simulink model "two_link_inner_loop"  (R2021a)
settings: Solver=VariableStepAuto  StartTime=0.0  StopTime=10.0  RelTol=1e-3
undefined symbols (not defined in the file): a_1, a_2, F, K, K_D, K_F, K_P, M_d, o_r
settings Model: Creator=frida  LastModifiedBy=frida

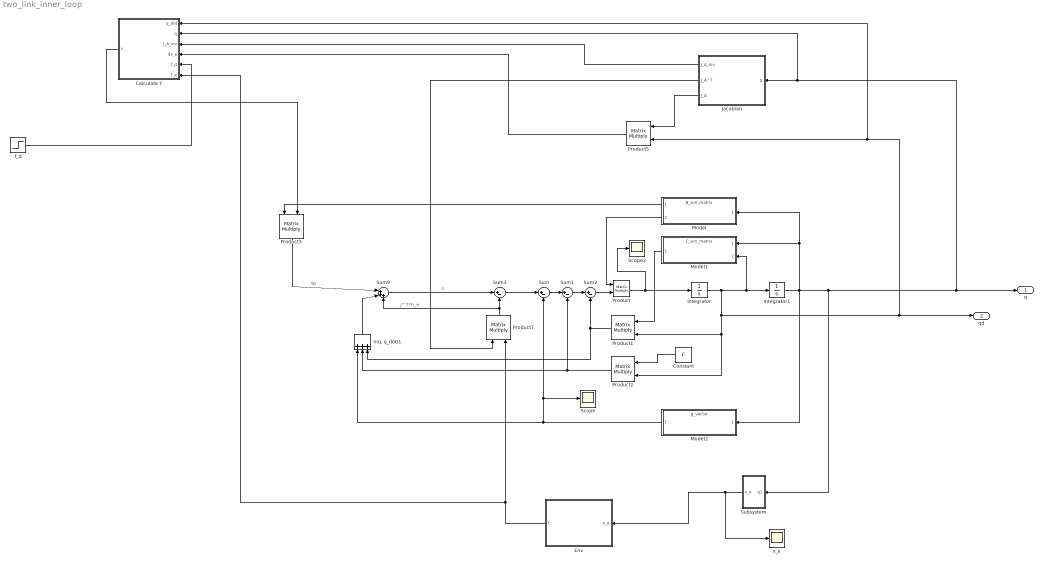
== system two_link_inner_loop ==
  note: J^T*h_e
  Calculate Y : Subsystem
  Constant : Constant  Value=F
  Env : Subsystem
  Integrator : Integrator
  Integrator1 : Integrator  InitialCondition=[0.75*pi, -0.75*pi]
  Jacobian : Subsystem
  Model : ModelReference  ModelNameDialog=B_sim_matrix.slx  SimulationMode=Normal  ModelReferenceVersion=1.6
  Model1 : ModelReference  ModelNameDialog=C_sim_matrix.slx  SimulationMode=Normal  ModelReferenceVersion=1.2
  Model2 : ModelReference  ModelNameDialog=g_vector.slx  SimulationMode=Normal  ModelReferenceVersion=1.8
  Product{,1..3,5,7} (6 alike) : Product  Multiplication=Matrix(*)
  Scope : Scope
  Scope2 : Scope
  Subsystem : Subsystem
  Sum{,1..3} (4 alike) : Sum  Inputs=|+-
  Sum9 : Sum  Inputs=|+++
  f_d : Step  After=[5,0]  SampleTime=0
  "n(q, q_dot)1" : Sum  Inputs=+++
  x_e : Scope
  q : Outport  PortDimensions=2
  qd : Outport  Port=2  PortDimensions=2
  wires:
  Constant/1 -> Product2/1
  Integrator/1 -> Calculate Y/1(q_dot), Product5/2, qd/1, Product2/2, Product1/2, Model1/2, Integrator1/1
  Sum3/1 -> Sum/1
  Product/1 -> Integrator/1, Scope2/1
  Jacobian/2(J_A^T) -> Product7/1
  Calculate Y/1(Y) -> Product3/2
  Jacobian/1(J_A_inv) -> Calculate Y/3(J_A_inv)
  Model2/1 -> "n(q, q_dot)1"/1, Scope/1, Sum/2
  Sum/1 -> Sum1/1
  Product7/1 -> Sum3/2, Sum9/3
  Model1/1 -> Product1/1
  Sum2/1 -> Product/2
  "n(q, q_dot)1"/1 -> Sum9/2
  Product5/1 -> Calculate Y/4(dx_e)
  Model/1 -> Product3/1
  Env/1(f) -> Calculate Y/6(f_e), Product7/2
  Jacobian/3(J_A) -> Product5/1
  Product3/1 -> Sum9/1  "By"
  Model/2 -> Product/1
  Integrator1/1 -> Model2/1, Calculate Y/2(q), Jacobian/1(q), q/1, Subsystem/1(q1), Model/1, Model1/1
  Sum9/1 -> Sum3/1  "U"
  Product2/1 -> "n(q, q_dot)1"/2, Sum1/2
  Subsystem/1(o_e) -> x_e/1, Env/1(o_e)
  Product1/1 -> "n(q, q_dot)1"/3, Sum2/2
  Sum1/1 -> Sum2/1
  f_d/1 -> Calculate Y/5(f_d)

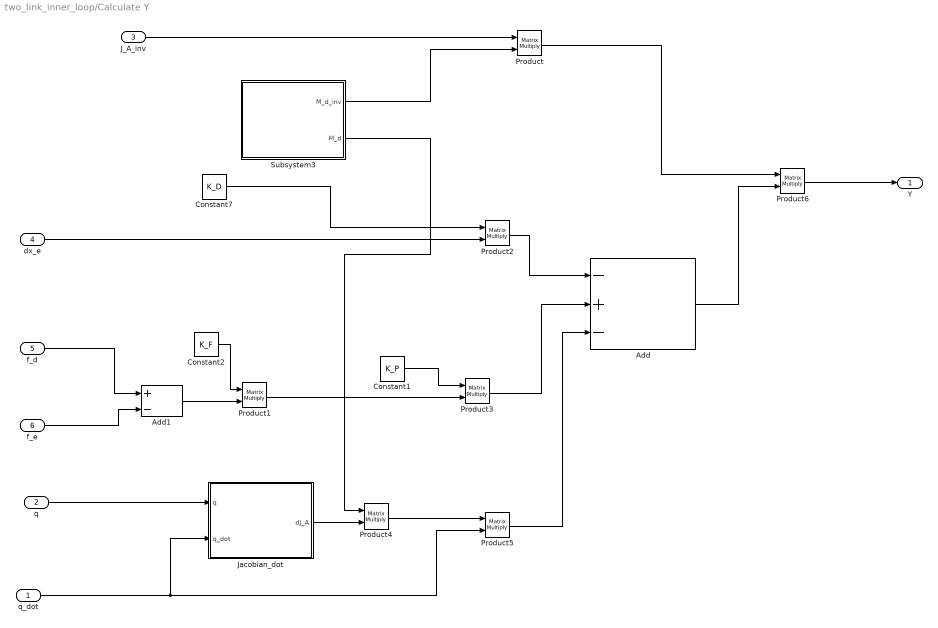
== system two_link_inner_loop/Calculate Y ==
  q_dot : Inport
  q : Inport  Port=2
  J_A_inv : Inport  Port=3
  dx_e : Inport  Port=4
  f_d : Inport  Port=5
  f_e : Inport  Port=6
  Add : Sum  Inputs=-+-
  Add1 : Sum  Inputs=+-
  Constant1 : Constant  Value=K_P
  Constant2 : Constant  Value=K_F
  Constant7 : Constant  Value=K_D
  Jacobian_dot : Subsystem
  Product{,1..6} (7 alike) : Product  Multiplication=Matrix(*)
  Subsystem3 : Subsystem
  Y : Outport
  wires:
  J_A_inv/1 -> Product/1
  Subsystem3/1(M_d_inv) -> Product/2
  Subsystem3/2(M_d) -> Product4/1
  Constant7/1 -> Product2/1
  Product2/1 -> Add/1
  Constant1/1 -> Product3/1
  Product3/1 -> Add/2
  Jacobian_dot/1(dJ_A) -> Product4/2
  Product4/1 -> Product5/1
  Product5/1 -> Add/3
  q/1 -> Jacobian_dot/1(q)
  q_dot/1 -> Product5/2, Jacobian_dot/2(q_dot)
  Product/1 -> Product6/1
  Add/1 -> Product6/2
  Product6/1 -> Y/1
  dx_e/1 -> Product2/2
  Constant2/1 -> Product1/1
  f_d/1 -> Add1/1
  f_e/1 -> Add1/2
  Add1/1 -> Product1/2
  Product1/1 -> Product3/2

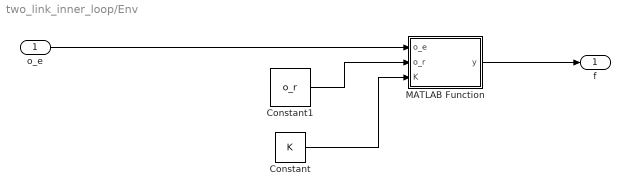
== system two_link_inner_loop/Env ==
  o_e : Inport
  Constant : Constant  Value=K
  Constant1 : Constant  Value=o_r
  MATLAB Function : MATLAB Function  TreatAsAtomicUnit=on
  f : Outport
  wires:
  Constant1/1 -> MATLAB Function/2(o_r)
  Constant/1 -> MATLAB Function/3(K)
  MATLAB Function/1(y) -> f/1
  o_e/1 -> MATLAB Function/1(o_e)

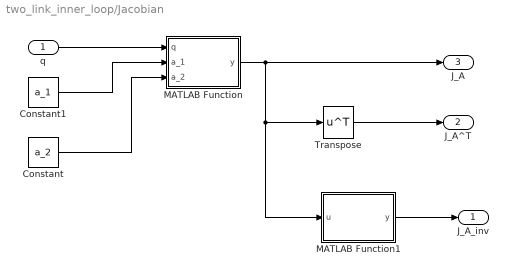
== system two_link_inner_loop/Jacobian ==
  q : Inport
  Constant : Constant  Value=a_2
  Constant1 : Constant  Value=a_1
  MATLAB Function : MATLAB Function  TreatAsAtomicUnit=on
  MATLAB Function1 : MATLAB Function  TreatAsAtomicUnit=on
  Transpose : Math  Operator=transpose  SaturateOnIntegerOverflow=on
  J_A_inv : Outport
  J_A^T : Outport  Port=2
  J_A : Outport  Port=3
  wires:
  MATLAB Function/1(y) -> MATLAB Function1/1(u), Transpose/1, J_A/1
  q/1 -> MATLAB Function/1(q)
  Constant1/1 -> MATLAB Function/2(a_1)
  Constant/1 -> MATLAB Function/3(a_2)
  Transpose/1 -> J_A^T/1
  MATLAB Function1/1(y) -> J_A_inv/1

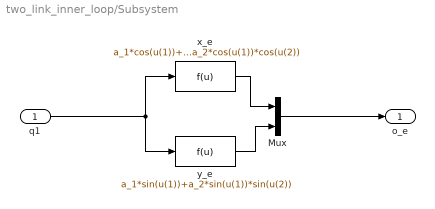
== system two_link_inner_loop/Subsystem ==
  q1 : Inport
  Mux : Mux  Inputs=2
  x_e : Fcn  Expr=a_1*cos(u(1))+a_2*cos(u(1))*cos(u(2))
  y_e : Fcn  Expr=a_1*sin(u(1))+a_2*sin(u(1))*sin(u(2))
  o_e : Outport
  wires:
  x_e/1 -> Mux/1
  Mux/1 -> o_e/1
  y_e/1 -> Mux/2
  q1/1 -> y_e/1, x_e/1

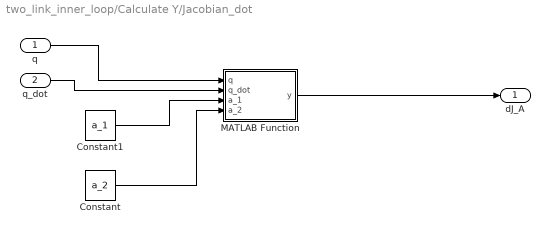
== system two_link_inner_loop/Calculate Y/Jacobian_dot ==
  q : Inport
  q_dot : Inport  Port=2
  Constant : Constant  Value=a_2
  Constant1 : Constant  Value=a_1
  MATLAB Function : MATLAB Function  TreatAsAtomicUnit=on
  dJ_A : Outport
  wires:
  MATLAB Function/1(y) -> dJ_A/1
  q/1 -> MATLAB Function/1(q)
  Constant1/1 -> MATLAB Function/3(a_1)
  Constant/1 -> MATLAB Function/4(a_2)
  q_dot/1 -> MATLAB Function/2(q_dot)

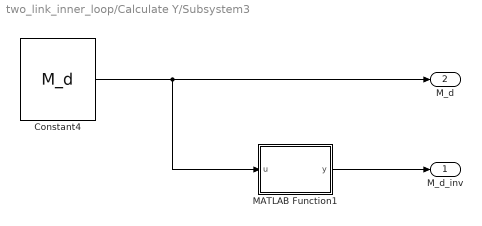
== system two_link_inner_loop/Calculate Y/Subsystem3 ==
  Constant4 : Constant  Value=M_d
  MATLAB Function1 : MATLAB Function  TreatAsAtomicUnit=on
  M_d_inv : Outport
  M_d : Outport  Port=2
  wires:
  Constant4/1 -> MATLAB Function1/1(u), M_d/1
  MATLAB Function1/1(y) -> M_d_inv/1

== matlab function two_link_inner_loop/Jacobian/MATLAB Function ==
  data: q input; y output; a_1 input; a_2 input
function y = fcn(q, a_1, a_2)
y = [-a_1*sin(q(1)) - a_2*sin(q(1))*sin(q(2)), -a_2*sin(q(1))*sin(q(2));
    a_1*cos(q(1)) + a_2*cos(q(1))*cos(q(2)), a_2*cos(q(1))*cos(q(2))];

== matlab function two_link_inner_loop/Env/MATLAB Function ==
  data: o_e input; y output; o_r input; K input
function y = fcn(o_e, o_r, K)
if o_e(1) < o_r(1)
    y = [0; 0];
else
    % In this case the K matrix is a 
    % (2 x 2) matrix where only k_x is defined, 
    % therefore the returned y contains 
    % only forces in x-direction
    y = K*[o_e(1)-o_r(1); o_e(2)-o_r(2)];
end

== matlab function two_link_inner_loop/Jacobian/MATLAB Function1 ==
  data: u input; y output
function y = fcn(u)
%#codegen

y = inv(u);

== matlab function two_link_inner_loop/Calculate Y/Jacobian_dot/MATLAB Function ==
  data: q input; q_dot input; y output; a_1 input; a_2 input
function y = fcn(q, q_dot, a_1, a_2)
y = [-a_1*cos(q(1))*q_dot(1) - a_2*sin(q(1))*cos(q(2))*q_dot(2) - a_2*sin(q(2))*cos(q(1))*q_dot(1), -a_2*sin(q(1))*cos(q(2))*q_dot(2) + sin(q(2))*cos(q(1))*q_dot(1);
    -a_1*sin(q(1))*q_dot(1) - a_2*sin(q(1))*cos(q(2))*q_dot(1) - a_2*sin(q(2))*cos(q(1))*q_dot(2), -a_2*sin(q(1))*cos(q(2))*q_dot(1) + sin(q(2))*cos(q(1))*q_dot(2)];

== matlab function two_link_inner_loop/Calculate Y/Subsystem3/MATLAB Function1 ==
  data: u input; y output
function y = fcn(u)
%#codegen

y = inv(u);
